simulink model "Control_model_10DOF_fin"  (R2016b)
settings: Solver=FixedStepAuto  StartTime=0.0  StopTime=10  FixedStep=0.0001  RelTol=1e-3
InitFcn:
  | Initialisation_ctr_10DOF_fin
values from neighbouring files (symbols this model uses):
  COM_Parameters = [-lpelvis/2;r2;0]    [Initialisation_ctr_10DOF_fin.m]
  DH_Parameters = [hfoot 0 ... (first row only)    [Initialisation_ctr_10DOF_fin.m]
  dTrunk = trunklbd(3)    [Initialisation_ctr_10DOF_fin.m]
  dxFootSM = dxFoot    [Initialisation_ctr_10DOF_fin.m]
  dxTrunk = 0.1    [Initialisation_ctr_10DOF_fin.m]
  Foot_Parameters = [0;-(lFoot/2-lHeel);0]    [Initialisation_ctr_10DOF_fin.m]
  HAA2HEE = [0; 0; 0.001]    [Initialisation_ctr_10DOF_fin.m]
  HEE2HFE = 0.5*[0.2; 0; 0]    [Initialisation_ctr_10DOF_fin.m]
  height_vrp = CoM_position(1)    [Initialisation_ctr_10DOF_fin.m]
  hTrunk = trunklbd(1)    [Initialisation_ctr_10DOF_fin.m]
  initial_CoM_position = R*CoM_position    [Initialisation_ctr_10DOF_fin.m]
  initial_CoM_velocity = [0;0;0]    [Initialisation_ctr_10DOF_fin.m]
  initial_left_foot = [0;0;-stance_width/2]    [Initialisation_ctr_10DOF_fin.m]
  initial_right_foot = [0;0;stance_width/2]    [Initialisation_ctr_10DOF_fin.m]
  initial_RorL = 0    [Initialisation_ctr_10DOF_fin.m]
  jointsinitial = [9;-15;6;0;0;6;-15;9]/180*pi    [Initialisation_ctr_10DOF_fin.m]
  K_DCM = 4.3*[1 0 0 ... (first row only)    [Initialisation_ctr_10DOF_fin.m]
  kD_left = mbody*[0.95 0 0 0 ... (first row only)    [Initialisation_ctr_10DOF_fin.m]
  kD_right = mbody*[0.12 0 0 0 ... (first row only)    [Initialisation_ctr_10DOF_fin.m]
  kI_left = mbody*[35 0 0 0 ... (first row only)    [Initialisation_ctr_10DOF_fin.m]
  kI_right = mbody*[38.2 0 0 0 ... (first row only)    [Initialisation_ctr_10DOF_fin.m]
  kP_left = mbody*[75 0 0 0 ... (first row only)    [Initialisation_ctr_10DOF_fin.m]
  kP_right = mbody*[5.6 0 0 0 ... (first row only)    [Initialisation_ctr_10DOF_fin.m]
  Lenght = [lShank;lThigh]    [Initialisation_ctr_10DOF_fin.m]
  lFootSM = lFoot    [Initialisation_ctr_10DOF_fin.m]
  lpelvis = wPelvis    [Initialisation_ctr_10DOF_fin.m]
  mass = mbody    (= 60)    [Initialisation_ctr_10DOF_fin.m]
  Masses = [mThigh; mShank; mTrunk]    [Initialisation_ctr_10DOF_fin.m]
  nb_step = 4    [Initialisation_ctr_10DOF_fin.m]
  nb_step_pattern = 20    [Initialisation_ctr_10DOF_fin.m]
  Pelvis_Parameters = [-lpelvis/2;hTrunk/2;0]    [Initialisation_ctr_10DOF_fin.m]
  stance_width = lpelvis    [Initialisation_ctr_10DOF_fin.m]
  stride_lenght = 0.50    (= 0.5)    [Initialisation_ctr_10DOF_fin.m]
  T_DS = time_DS    (= 0.4)    [Initialisation_ctr_10DOF_fin.m]
  T_IT = time_DS    (= 0.4)    [Initialisation_ctr_10DOF_fin.m]
  T_SS = time_swing    (= 1.6)    [Initialisation_ctr_10DOF_fin.m]
  time_DS = (time_stance-time_swing)/2    (= 0.4)    [Initialisation_ctr_10DOF_fin.m]
  time_stance = 60/100*time_stride    (= 2.4)    [Initialisation_ctr_10DOF_fin.m]
  time_step = time_stride/2    (= 2)    [Initialisation_ctr_10DOF_fin.m]
  time_swing = 40/100*time_stride    (= 1.6)    [Initialisation_ctr_10DOF_fin.m]
  validity_angle = [-20*pi/180 20*pi/180 ... (first row only)    [Initialisation_ctr_10DOF_fin.m]
  wTrunk = trunklbd(2)    [Initialisation_ctr_10DOF_fin.m]
  x4CoM = CoM_position(1)-XR4(1)    [Initialisation_ctr_10DOF_fin.m]
undefined symbols (not defined in the file or in its folder): dsegment, hFoot, l, lFoot, omega0_x, omega0_z, rho, wPelvis, X, Xp_x, Xp_z, Y, Z
undefined symbols (not defined in the file): k_grf, lShankSM, lThighSM, mShank, mThigh
libraries: nesl_utility x247, sm_lib x215, dspindex x12, FootPlacementLibrary x8, dspsigops x4, dspswit3 x1
(part 6 of 18)

== system Control_model_10DOF_fin/10DoF Walker SimMechanics Model/Graphic/extrapolated CoM1 ==
  Foot_adjust : Inport
  Cartesian Joint : sm_lib/Joints/Cartesian Joint  SenseConstraintForce=off  SenseConstraintForceX=off  SenseConstraintForceY=off  SenseConstraintForceZ=off  SenseConstraintTorque=off  SenseConstraintTorqueX=off  SenseConstraintTorqueY=off  SenseConstraintTorqueZ=off  SenseTotalForce=off  SenseTotalForceX=off  SenseTotalForceY=off  SenseTotalForceZ=off  SenseTotalTorque=off  SenseTotalTorqueX=off  SenseTotalTorqueY=off  SenseTotalTorqueZ=off  CompositeWrenchDir=FollowerOnBase  CompositeWrenchFrame=BaseFrame  PxEquilibriumPosition=0  PxEquilibriumPositionUnits=m  PxSpringStiffness=0  PxSpringStiffnessUnits=N/m  PxDampingCoefficient=0  PxDampingCoefficientUnits=N/(m/s)  PxTorqueActuationMode=ComputedTorque  PxMotionActuationMode=InputMotion  PxSensePosition=off  PxSenseVelocity=off  PxSenseAcceleration=off  PxSenseTorqueForce=off  PxPositionTargetSpecify=on  PxPositionTargetPriority=Low  PxPositionTargetValue=0  PxPositionTargetValueUnits=m  PxVelocityTargetSpecify=off  PxVelocityTargetPriority=High  PxVelocityTargetValue=0  PxVelocityTargetValueUnits=m/s  PyEquilibriumPosition=0  PyEquilibriumPositionUnits=m  PySpringStiffness=0  PySpringStiffnessUnits=N/m  PyDampingCoefficient=0  PyDampingCoefficientUnits=N/(m/s)  PyTorqueActuationMode=ComputedTorque  PyMotionActuationMode=InputMotion  PySensePosition=off  PySenseVelocity=off  PySenseAcceleration=off  PySenseTorqueForce=off  PyPositionTargetSpecify=on  PyPositionTargetPriority=Low  PyPositionTargetValue=0  PyPositionTargetValueUnits=m  PyVelocityTargetSpecify=off  PyVelocityTargetPriority=High  PyVelocityTargetValue=0  PyVelocityTargetValueUnits=m/s  PzEquilibriumPosition=0  PzEquilibriumPositionUnits=m  PzSpringStiffness=0  PzSpringStiffnessUnits=N/m  PzDampingCoefficient=0  PzDampingCoefficientUnits=N/(m/s)  PzTorqueActuationMode=ComputedTorque  PzMotionActuationMode=InputMotion  PzSensePosition=off  PzSenseVelocity=off  PzSenseAcceleration=off  PzSenseTorqueForce=off  PzPositionTargetSpecify=on  PzPositionTargetPriority=Low  PzPositionTargetValue=0  PzPositionTargetValueUnits=m  PzVelocityTargetSpecify=off  PzVelocityTargetPriority=High  PzVelocityTargetValue=0  PzVelocityTargetValueUnits=m/s
  Demux : Demux  Outputs=3
  Graphic : sm_lib/Body Elements/Graphic  GraphicType=Marker  MarkerShape=Sphere  MarkerSize=10  GraphicVisPropType=SimpleVisualProperties  GraphicDiffuseColor=[0.0 0.2 0.4]  GraphicSpecularColor=[0.5 0.5 0.5 1.0]  GraphicAmbientColor=[0.15 0.15 0.15 1.0]  GraphicEmissiveColor=[0.0 0.0 0.0 1.0]  GraphicShininess=75  GraphicOpacity=1.0
  Memory2 : Memory  X0=[0;0;0]
  Rigid Transform1 : sm_lib/Frames and Transforms/Rigid Transform  TranslationMethod=None  TranslationStandardOffset=0  TranslationLengthUnit=m  TranslationStandardAxis=+Z  TranslationCartesianOffset=[0 0 0]  TranslationROffset=0  TranslationROffsetUnits=m  TranslationZOffset=0  TranslationZOffsetUnits=m  TranslationThetaOffset=0  TranslationThetaOffsetUnits=deg  RotationMethod=None  RotationAngleUnits=deg  RotationStandardAxis=+Z  RotationAngle=0.0  RotationArbitraryAxis=[0 0 1]  FollAlignAxisA=+X  BaseAlignAxisA=+Y  FollAlignAxisB=+Y  BaseAlignAxisB=+Z  RotationSequenceAxes=FollowerAxes  RotationSequence=XYX  RotationSequenceAngles=[0 0 0]  RotationSequenceAnglesUnits=deg  RotationMatrix=[1 0 0; 0 1 0; 0 0 1]
  Simulink-PS Converter1 : nesl_utility/Simulink-PS Converter  PhysicalDomain=network_engine_domain  SubClassName=ps_input  LeftPortType=input  RightPortType=output  PseudoPeriodic=off  Frequencies=[]  NoiseDistribution=none  NoiseParameters=[]  Unit=m  AffineConversion=on  InputFiltering=off  SimscapeFilterOrder=1  InputFilterTimeConstant=0.001  UdotUserProvided=1
  Simulink-PS Converter2 : nesl_utility/Simulink-PS Converter  PhysicalDomain=network_engine_domain  SubClassName=ps_input  LeftPortType=input  RightPortType=output  PseudoPeriodic=off  Frequencies=[]  NoiseDistribution=none  NoiseParameters=[]  Unit=m  AffineConversion=on  InputFiltering=off  SimscapeFilterOrder=1  InputFilterTimeConstant=0.001  UdotUserProvided=1
  Simulink-PS Converter7 : nesl_utility/Simulink-PS Converter  PhysicalDomain=network_engine_domain  SubClassName=ps_input  LeftPortType=input  RightPortType=output  PseudoPeriodic=off  Frequencies=[]  NoiseDistribution=none  NoiseParameters=[]  Unit=m  AffineConversion=on  InputFiltering=off  SimscapeFilterOrder=1  InputFilterTimeConstant=0.001  UdotUserProvided=1
  Base : PMIOPort  Port=1  Side=Left
  wires:
  Demux/1 -> Simulink-PS Converter7/1
  Demux/2 -> Simulink-PS Converter1/1
  Demux/3 -> Simulink-PS Converter2/1
  Memory2/1 -> Demux/1
  Foot_adjust/1 -> Memory2/1
  connections:
  Rigid Transform1/LConn1 -- Cartesian Joint/RConn1
  Simulink-PS Converter7/RConn1 -- Cartesian Joint/LConn2
  Rigid Transform1/RConn1 -- Graphic/RConn1
  Simulink-PS Converter1/RConn1 -- Cartesian Joint/LConn3
  Simulink-PS Converter2/RConn1 -- Cartesian Joint/LConn4
  Base/RConn1 -- Cartesian Joint/LConn1

== system Control_model_10DOF_fin/10DoF Walker SimMechanics Model/trunk/Forward Initial Velocity ==
  PelvisForceVector : Inport
  Perturbation : Inport  Port=2
  6-DOF Joint : sm_lib/Joints/6-DOF Joint  SenseConstraintForce=off  SenseConstraintForceX=off  SenseConstraintForceY=off  SenseConstraintForceZ=off  SenseConstraintTorque=off  SenseConstraintTorqueX=off  SenseConstraintTorqueY=off  SenseConstraintTorqueZ=off  SenseTotalForce=off  SenseTotalForceX=off  SenseTotalForceY=off  SenseTotalForceZ=off  SenseTotalTorque=off  SenseTotalTorqueX=off  SenseTotalTorqueY=off  SenseTotalTorqueZ=off  CompositeWrenchDir=FollowerOnBase  CompositeWrenchFrame=BaseFrame  PxEquilibriumPosition=0  PxEquilibriumPositionUnits=m  PxSpringStiffness=0  PxSpringStiffnessUnits=N/m  PxDampingCoefficient=0  PxDampingCoefficientUnits=N/(m/s)  PxTorqueActuationMode=NoTorque  PxMotionActuationMode=ComputedMotion  PxSensePosition=off  PxSenseVelocity=off  PxSenseAcceleration=off  PxSenseTorqueForce=off  PxPositionTargetSpecify=off  PxPositionTargetPriority=High  PxPositionTargetValue=0  PxPositionTargetValueUnits=m  PxVelocityTargetSpecify=off  PxVelocityTargetPriority=Low  PxVelocityTargetValue=initial_CoM_velocity(1)  PxVelocityTargetValueUnits=m/s  PyEquilibriumPosition=0  PyEquilibriumPositionUnits=m  PySpringStiffness=0  PySpringStiffnessUnits=N/m  PyDampingCoefficient=0  PyDampingCoefficientUnits=N/(m/s)  PyTorqueActuationMode=NoTorque  PyMotionActuationMode=ComputedMotion  PySensePosition=off  PySenseVelocity=off  PySenseAcceleration=off  PySenseTorqueForce=off  PyPositionTargetSpecify=off  PyPositionTargetPriority=High  PyPositionTargetValue=0  PyPositionTargetValueUnits=m  PyVelocityTargetSpecify=off  PyVelocityTargetPriority=Low  PyVelocityTargetValue=initial_CoM_velocity(2)  PyVelocityTargetValueUnits=m/s  PzEquilibriumPosition=0  PzEquilibriumPositionUnits=m  PzSpringStiffness=0  PzSpringStiffnessUnits=N/m  PzDampingCoefficient=0  PzDampingCoefficientUnits=N/(m/s)  PzTorqueActuationMode=NoTorque  PzMotionActuationMode=ComputedMotion  PzSensePosition=off  PzSenseVelocity=off  PzSenseAcceleration=off  PzSenseTorqueForce=off  PzPositionTargetSpecify=off  PzPositionTargetPriority=High  PzPositionTargetValue=0  PzPositionTargetValueUnits=m  PzVelocityTargetSpecify=off  PzVelocityTargetPriority=Low  PzVelocityTargetValue=initial_CoM_velocity(3)  PzVelocityTargetValueUnits=m/s  SphDefPosRotationMethod=None  SphDefPosRotationAngleUnits=deg  SphDefPosRotationStandardAxis=+Z  SphDefPosRotationAngle=0  SphDefPosRotationArbitraryAxis=[0 0 1]  SphDefPosFollAlignAxisA=+X  SphDefPosBaseAlignAxisA=+Y  SphDefPosFollAlignAxisB=+Y  SphDefPosBaseAlignAxisB=+Z  SphDefPosRotationSequenceAxes=FollowerAxes  SphDefPosRotationSequence=XYX  SphDefPosRotationSequenceAngles=[0 0 0]  SphDefPosRotationSequenceAnglesUnits=deg  SphDefPosRotationMatrix=[1 0 0; 0 1 0; 0 0 1]  SphEqPosRotationMethod=StandardAxis  SphEqPosRotationAngleUnits=deg  SphEqPosRotationStandardAxis=+Y  SphEqPosRotationAngle=0  SphEqPosRotationArbitraryAxis=[0 0 1]  SphEqPosFollAlignAxisA=+X  SphEqPosBaseAlignAxisA=+Y  SphEqPosFollAlignAxisB=+Y  SphEqPosBaseAlignAxisB=+Z  SphEqPosRotationSequenceAxes=FollowerAxes  SphEqPosRotationSequence=XYX  SphEqPosRotationSequenceAngles=[0 0 0]  SphEqPosRotationSequenceAnglesUnits=deg  SphEqPosRotationMatrix=[1 0 0; 0 1 0; 0 0 1]  SphSpringStiffness=100  SphSpringStiffnessUnits=N*m/rad  SphDampingCoefficient=10  SphDampingCoefficientUnits=N*m/(rad/s)  SphActuateTorqueX=off  SphActuateTorqueY=off  SphActuateTorqueZ=off  SphActuateTorque=off  SphTorqueActuationMode=NoTorque  SphMotionActuationMode=ComputedMotion  SphActuationFrame=BaseFrame  SphSensePosition=off  SphSenseVelocityX=off  SphSenseVelocityY=off  SphSenseVelocityZ=off  SphSenseVelocity=off  SphSenseAccelerationX=off  SphSenseAccelerationY=off  SphSenseAccelerationZ=off  SphSenseAcceleration=off  SphSenseTorqueX=off  SphSenseTorqueY=off  SphSenseTorqueZ=off  SphSenseTorqueForce=off  SphSensingFrame=BaseFrame  SphPositionTargetRotationMethod=StandardAxis  SphPositionTargetRotationAngleUnits=deg  SphPositionTargetRotationStandardAxis=+X  SphPositionTargetRotationAngle=0  SphPositionTargetRotationArbitraryAxis=[0 0 1]  SphPositionTargetFollAlignAxisA=+X  SphPositionTargetBaseAlignAxisA=+Y  SphPositionTargetFollAlignAxisB=+Y  SphPositionTargetBaseAlignAxisB=+Z  SphPositionTargetRotationSequenceAxes=FollowerAxes  SphPositionTargetRotationSequence=XYX  SphPositionTargetRotationSequenceAngles=[0 0 0]  SphPositionTargetRotationSequenceAnglesUnits=deg  SphPositionTargetRotationMatrix=[1 0 0; 0 1 0; 0 0 1]  SphPositionTargetSpecify=off  SphPositionTargetPriority=Low  SphVelocityTargetValue=[0 0 0]  SphVelocityTargetValueUnits=deg/s  SphVelocityTargetSpecify=off  SphVelocityTargetPriority=High  SphVelocityTargetInFollowerFrame=on
  Demux : Demux  Outputs=3
  External Force  and Torque : sm_lib/Forces and Torques/External Force and Torque  ForceResolutionFrame=World  EnableForceX=off  EnableForceY=off  EnableForceZ=on  EnableForce=off  TorqueResolutionFrame=AttachedFrame  EnableTorqueX=off  EnableTorqueY=off  EnableTorqueZ=off  EnableTorque=off
  External Force  and Torque2 : sm_lib/Forces and Torques/External Force and Torque  ForceResolutionFrame=World  EnableForceX=on  EnableForceY=off  EnableForceZ=on  EnableForce=off  TorqueResolutionFrame=AttachedFrame  EnableTorqueX=off  EnableTorqueY=off  EnableTorqueZ=off  EnableTorque=off
  Mux : Mux  Inputs=3
  Mux1 : Mux  Inputs=3
  PS-Simulink Converter{1..7} (7 alike) : nesl_utility/PS-Simulink Converter  PhysicalDomain=network_engine_domain  SubClassName=ps_output  LeftPortType=input  RightPortType=output  PseudoPeriodic=off  Frequencies=[]  Unit=1  AffineConversion=off
  Simulink-PS Converter1 : nesl_utility/Simulink-PS Converter  PhysicalDomain=network_engine_domain  SubClassName=ps_input  LeftPortType=input  RightPortType=output  PseudoPeriodic=off  Frequencies=[]  NoiseDistribution=none  NoiseParameters=[]  Unit=N  AffineConversion=off  InputFiltering=off  SimscapeFilterOrder=1  InputFilterTimeConstant=0.001  UdotUserProvided=1
  Simulink-PS Converter3 : nesl_utility/Simulink-PS Converter  PhysicalDomain=network_engine_domain  SubClassName=ps_input  LeftPortType=input  RightPortType=output  PseudoPeriodic=off  Frequencies=[]  NoiseDistribution=none  NoiseParameters=[]  Unit=N  AffineConversion=off  InputFiltering=off  SimscapeFilterOrder=1  InputFilterTimeConstant=0.001  UdotUserProvided=1
  Terminator : Terminator
  Terminator1 : Terminator
  Transform  Sensor : sm_lib/Frames and Transforms/Transform Sensor  MeasurementFrame=Base  SenseAngle=off  SenseAxis=off  SenseAngle1=off  SenseAngle2=off  SenseAngle3=off  SenseQ=off  SenseR=off  SenseOmegaX=off  SenseOmegaY=off  SenseOmegaZ=off  SenseOmega1=off  SenseOmega2=off  SenseOmega3=off  SenseQDot=off  SenseRDot=off  SenseAlphaX=off  SenseAlphaY=off  SenseAlphaZ=off  SenseAlpha1=off  SenseAlpha2=off  SenseAlpha3=off  SenseQDDot=off  SenseRDDot=off  SenseX=off  SenseY=off  SenseZ=off  SenseRad=off  SenseAzim=off  SenseDist=off  SenseInc=off  SenseXDot=off  SenseYDot=off  SenseZDot=off  SenseRadDot=off  SenseAzimDot=off  SenseDistDot=off  SenseIncDot=off  SenseXDDot=on  SenseYDDot=on  SenseZDDot=on  SenseRadDDot=off  SenseAzimDDot=off  SenseDistDDot=off  SenseIncDDot=off
  Transform  Sensor1 : sm_lib/Frames and Transforms/Transform Sensor  MeasurementFrame=Base  SenseAngle=off  SenseAxis=off  SenseAngle1=off  SenseAngle2=off  SenseAngle3=off  SenseQ=off  SenseR=off  SenseOmegaX=off  SenseOmegaY=off  SenseOmegaZ=off  SenseOmega1=off  SenseOmega2=off  SenseOmega3=off  SenseQDot=off  SenseRDot=off  SenseAlphaX=off  SenseAlphaY=off  SenseAlphaZ=off  SenseAlpha1=off  SenseAlpha2=off  SenseAlpha3=off  SenseQDDot=off  SenseRDDot=off  SenseX=off  SenseY=off  SenseZ=off  SenseRad=off  SenseAzim=off  SenseDist=off  SenseInc=off  SenseXDot=on  SenseYDot=on  SenseZDot=on  SenseRadDot=off  SenseAzimDot=off  SenseDistDot=off  SenseIncDot=off  SenseXDDot=off  SenseYDDot=off  SenseZDDot=off  SenseRadDDot=off  SenseAzimDDot=off  SenseDistDDot=off  SenseIncDDot=off
  Transform  Sensor2 : sm_lib/Frames and Transforms/Transform Sensor  MeasurementFrame=World  SenseAngle=off  SenseAxis=off  SenseAngle1=off  SenseAngle2=off  SenseAngle3=off  SenseQ=off  SenseR=on  SenseOmegaX=off  SenseOmegaY=off  SenseOmegaZ=off  SenseOmega1=off  SenseOmega2=off  SenseOmega3=off  SenseQDot=off  SenseRDot=off  SenseAlphaX=off  SenseAlphaY=off  SenseAlphaZ=off  SenseAlpha1=off  SenseAlpha2=off  SenseAlpha3=off  SenseQDDot=off  SenseRDDot=off  SenseX=off  SenseY=off  SenseZ=off  SenseRad=off  SenseAzim=off  SenseDist=off  SenseInc=off  SenseXDot=off  SenseYDot=off  SenseZDot=off  SenseRadDot=off  SenseAzimDot=off  SenseDistDot=off  SenseIncDot=off  SenseXDDot=off  SenseYDDot=off  SenseZDDot=off  SenseRadDDot=off  SenseAzimDDot=off  SenseDistDDot=off  SenseIncDDot=off
  World : PMIOPort  Port=1  Side=Right
  PelvisCentre : PMIOPort  Port=2  Side=Right
  A_CoM : Outport
  V_CoM : Outport  Port=2
  Rtrunk : Outport  Port=3
  wires:
  PelvisForceVector/1 -> Demux/1
  PS-Simulink Converter3/1 -> Mux/1
  Mux/1 -> A_CoM/1
  PS-Simulink Converter1/1 -> Mux/2
  PS-Simulink Converter2/1 -> Mux/3
  PS-Simulink Converter4/1 -> Mux1/1
  Mux1/1 -> V_CoM/1
  PS-Simulink Converter5/1 -> Mux1/2
  PS-Simulink Converter6/1 -> Mux1/3
  PS-Simulink Converter7/1 -> Rtrunk/1
  Demux/3 -> Simulink-PS Converter1/1
  Perturbation/1 -> Simulink-PS Converter3/1
  Demux/1 -> Terminator/1
  Demux/2 -> Terminator1/1
  connections:
  6-DOF Joint/LConn1 -- Transform  Sensor1/LConn1 -- Transform  Sensor/LConn1 -- Transform  Sensor2/LConn1 -- World/RConn1
  6-DOF Joint/RConn1 -- Transform  Sensor2/RConn1 -- External Force  and Torque2/RConn1 -- External Force  and Torque/RConn1 -- Transform  Sensor1/RConn1 -- Transform  Sensor/RConn1 -- PelvisCentre/RConn1
  PS-Simulink Converter3/LConn1 -- Transform  Sensor/RConn2
  Simulink-PS Converter1/RConn1 -- External Force  and Torque/LConn1
  Transform  Sensor/RConn3 -- PS-Simulink Converter1/LConn1
  PS-Simulink Converter2/LConn1 -- Transform  Sensor/RConn4
  PS-Simulink Converter4/LConn1 -- Transform  Sensor1/RConn2
  PS-Simulink Converter5/LConn1 -- Transform  Sensor1/RConn3
  PS-Simulink Converter6/LConn1 -- Transform  Sensor1/RConn4
  PS-Simulink Converter7/LConn1 -- Transform  Sensor2/RConn2
  Simulink-PS Converter3/RConn1 -- External Force  and Torque2/LConn1

== system Control_model_10DOF_fin/10DoF Walker SimMechanics Model/trunk/Scope x3 ==
  Input : Inport
  Demux : Demux  Outputs=3
  Scope1 : Scope
  Scope2 : Scope
  Scope3 : Scope
  wires:
  Input/1 -> Demux/1
  Demux/2 -> Scope1/1
  Demux/3 -> Scope2/1
  Demux/1 -> Scope3/1

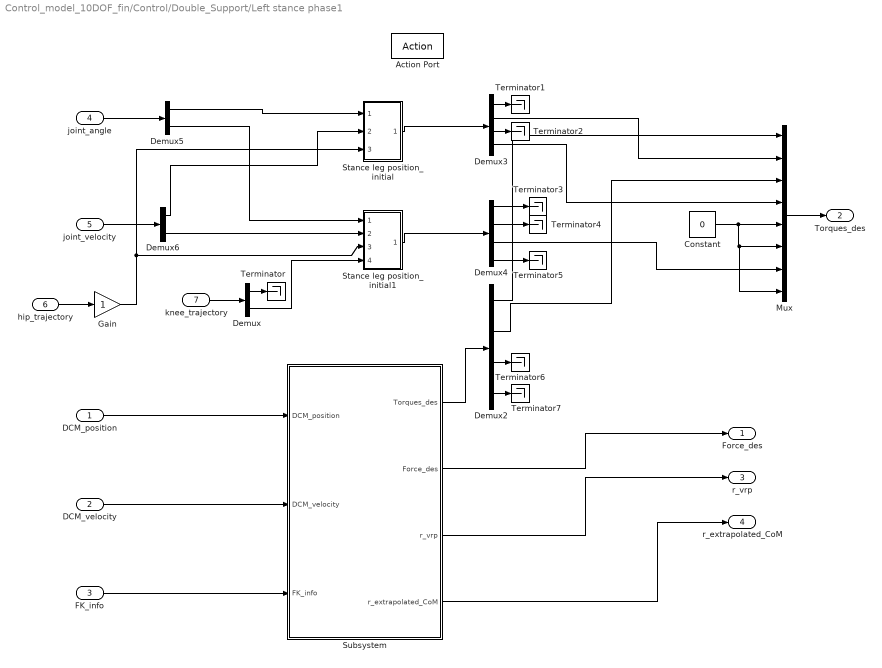
== system Control_model_10DOF_fin/Control/Double_Support/Left stance phase1 ==
  DCM_position : Inport
  DCM_velocity : Inport  Port=2
  FK_info : Inport  Port=3
  joint_angle : Inport  Port=4
  joint_velocity : Inport  Port=5
  hip_trajectory : Inport  Port=6
  knee_trajectory : Inport  Port=7
  Action Port : ActionPort  ActionType=else
  Constant : Constant  Value=0
  Demux : Demux  Outputs=2
  Demux2 : Demux
  Demux3 : Demux
  Demux4 : Demux
  Demux5 : Demux  Outputs=2
  Demux6 : Demux  Outputs=2
  Gain : Gain
  Mux : Mux  Inputs=8
  Stance leg position_initial : Subsystem
  Stance leg position_initial1 : Subsystem
  Subsystem : Subsystem
  Terminator{,1..7} (8 alike) : Terminator
  Force_des : Outport
  Torques_des : Outport  Port=2  OutDataTypeStr=double  Unit=N*m
  r_vrp : Outport  Port=3
  r_extrapolated_CoM : Outport  Port=4
  wires:
  joint_angle/1 -> Demux5/1
  joint_velocity/1 -> Demux6/1
  Subsystem/1(Torques_des) -> Demux2/1
  Mux/1 -> Torques_des/1
  Stance leg position_initial/1(torques) -> Demux3/1
  Stance leg position_initial1/1(torques) -> Demux4/1
  Demux5/1 -> Stance leg position_initial/1(position)
  Demux5/2 -> Stance leg position_initial1/1(position)
  Demux6/2 -> Stance leg position_initial1/2(velocity)
  Demux6/1 -> Stance leg position_initial/2(velocity)
  Subsystem/2(Force_des) -> Force_des/1
  Subsystem/3(r_vrp) -> r_vrp/1
  Subsystem/4(r_extrapolated_CoM) -> r_extrapolated_CoM/1
  Demux3/2 -> Mux/2
  Demux3/4 -> Mux/4
  DCM_position/1 -> Subsystem/1(DCM_position)
  FK_info/1 -> Subsystem/3(FK_info)
  DCM_velocity/1 -> Subsystem/2(DCM_velocity)
  hip_trajectory/1 -> Gain/1
  Gain/1 -> Stance leg position_initial/3(theta4), Stance leg position_initial1/3(theta5)
  Demux2/2 -> Mux/3
  Demux2/1 -> Mux/1
  Demux4/3 -> Mux/7
  knee_trajectory/1 -> Demux/1
  Demux/2 -> Stance leg position_initial1/4(knee_trajectory)
  Demux/1 -> Terminator/1
  Demux3/1 -> Terminator1/1
  Demux3/3 -> Terminator2/1
  Demux4/1 -> Terminator3/1
  Demux4/2 -> Terminator4/1
  Demux4/4 -> Terminator5/1
  Demux2/3 -> Terminator6/1
  Demux2/4 -> Terminator7/1
  Constant/1 -> Mux/8, Mux/6, Mux/5

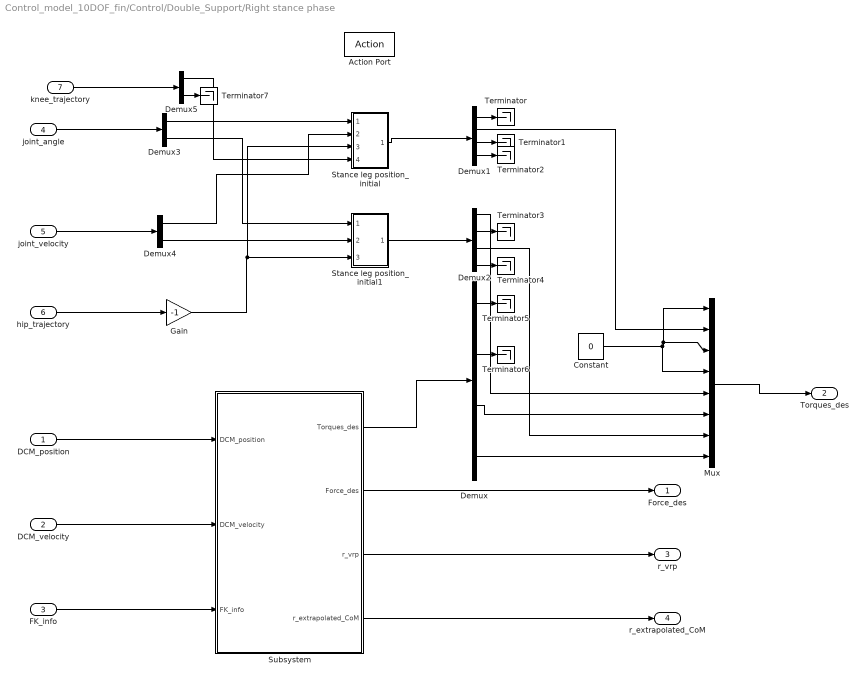
== system Control_model_10DOF_fin/Control/Double_Support/Right stance phase ==
  DCM_position : Inport
  DCM_velocity : Inport  Port=2
  FK_info : Inport  Port=3
  joint_angle : Inport  Port=4
  joint_velocity : Inport  Port=5
  hip_trajectory : Inport  Port=6
  knee_trajectory : Inport  Port=7
  Action Port : ActionPort  ActionType=then
  Constant : Constant  Value=0
  Demux : Demux
  Demux1 : Demux
  Demux2 : Demux
  Demux3 : Demux  Outputs=2
  Demux4 : Demux  Outputs=2
  Demux5 : Demux  Outputs=2
  Gain : Gain  Gain=-1
  Mux : Mux  Inputs=8
  Stance leg position_initial : Subsystem
  Stance leg position_initial1 : Subsystem
  Subsystem : Subsystem
  Terminator{,1..7} (8 alike) : Terminator
  Force_des : Outport
  Torques_des : Outport  Port=2  OutDataTypeStr=double  Unit=N*m
  r_vrp : Outport  Port=3
  r_extrapolated_CoM : Outport  Port=4
  wires:
  DCM_position/1 -> Subsystem/1(DCM_position)
  DCM_velocity/1 -> Subsystem/2(DCM_velocity)
  FK_info/1 -> Subsystem/3(FK_info)
  Subsystem/2(Force_des) -> Force_des/1
  Subsystem/3(r_vrp) -> r_vrp/1
  Subsystem/4(r_extrapolated_CoM) -> r_extrapolated_CoM/1
  Subsystem/1(Torques_des) -> Demux/1
  Stance leg position_initial/1(torques) -> Demux1/1
  Mux/1 -> Torques_des/1
  Stance leg position_initial1/1(torques) -> Demux2/1
  Demux3/1 -> Stance leg position_initial/1(position)
  Demux3/2 -> Stance leg position_initial1/1(position)
  Demux4/2 -> Stance leg position_initial1/2(velocity)
  Demux4/1 -> Stance leg position_initial/2(velocity)
  joint_angle/1 -> Demux3/1
  joint_velocity/1 -> Demux4/1
  Demux2/3 -> Mux/7
  Demux2/1 -> Mux/5
  Demux/3 -> Mux/6
  Demux/4 -> Mux/8
  hip_trajectory/1 -> Gain/1
  Gain/1 -> Stance leg position_initial/3(theta4), Stance leg position_initial1/3(theta5)
  knee_trajectory/1 -> Demux5/1
  Demux5/1 -> Stance leg position_initial/4(knee_trajectory)
  Demux1/2 -> Mux/2
  Demux1/1 -> Terminator/1
  Demux1/3 -> Terminator1/1
  Demux1/4 -> Terminator2/1
  Demux2/2 -> Terminator3/1
  Demux2/4 -> Terminator4/1
  Demux/1 -> Terminator5/1
  Demux/2 -> Terminator6/1
  Constant/1 -> Mux/4, Mux/3, Mux/1
  Demux5/2 -> Terminator7/1

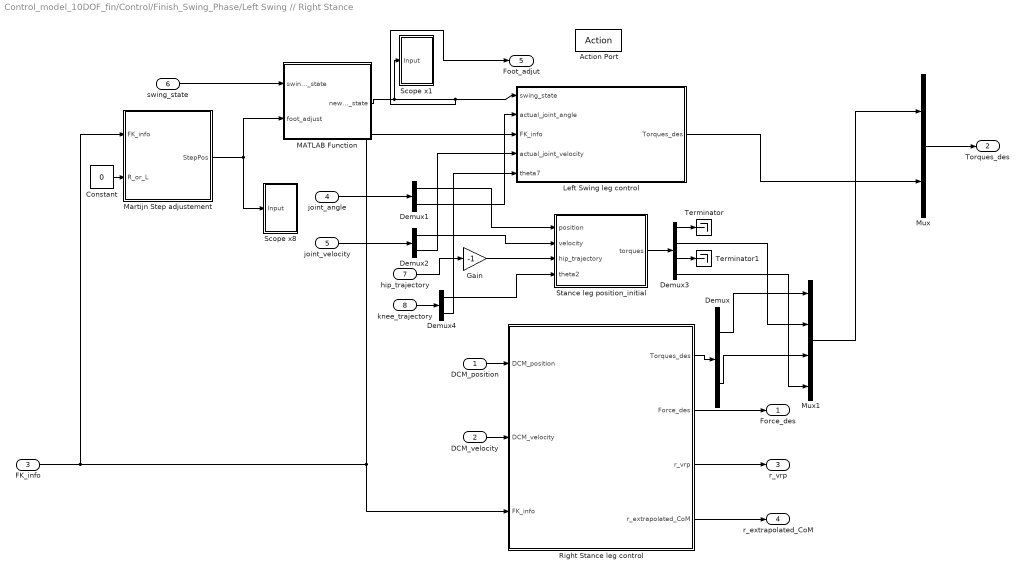
== system Control_model_10DOF_fin/Control/Finish_Swing_Phase/Left Swing // Right Stance ==
  DCM_position : Inport
  DCM_velocity : Inport  Port=2
  FK_info : Inport  Port=3
  joint_angle : Inport  Port=4
  joint_velocity : Inport  Port=5
  swing_state : Inport  Port=6
  hip_trajectory : Inport  Port=7
  knee_trajectory : Inport  Port=8
  Action Port : ActionPort  ActionType=then
  Constant : Constant  Value=0
  Demux{,1..2,4} (4 alike) : Demux  Outputs=2
  Demux3 : Demux
  Gain : Gain  Gain=-1
  Left Swing leg control : Subsystem
  MATLAB Function : MATLAB Function  TreatAsAtomicUnit=on
  Martijn Step adjustement : Subsystem
  Mux : Mux  Inputs=2
  Mux1 : Mux
  Right Stance leg control : Subsystem
  Scope x1 : Subsystem
  Scope x8 : Subsystem
  Stance leg position_initial : Subsystem
  Terminator : Terminator
  Terminator1 : Terminator
  Force_des : Outport
  Torques_des : Outport  Port=2  OutDataTypeStr=double  Unit=N*m
  r_vrp : Outport  Port=3
  r_extrapolated_CoM : Outport  Port=4
  Foot_adjut : Outport  Port=5
  wires:
  Left Swing leg control/1(Torques_des) -> Mux/2
  Right Stance leg control/1(Torques_des) -> Demux/1
  Stance leg position_initial/1(torques) -> Demux3/1
  Demux3/2 -> Mux1/2
  Right Stance leg control/2(Force_des) -> Force_des/1
  Mux/1 -> Torques_des/1
  Right Stance leg control/4(r_extrapolated_CoM) -> r_extrapolated_CoM/1
  Right Stance leg control/3(r_vrp) -> r_vrp/1
  FK_info/1 -> Left Swing leg control/3(FK_info), Right Stance leg control/3(FK_info), Martijn Step adjustement/1(FK_info)
  DCM_velocity/1 -> Right Stance leg control/2(DCM_velocity)
  DCM_position/1 -> Right Stance leg control/1(DCM_position)
  Demux1/1 -> Stance leg position_initial/1(position)
  Demux1/2 -> Left Swing leg control/2(actual_joint_angle)
  joint_angle/1 -> Demux1/1
  joint_velocity/1 -> Demux2/1
  Demux2/1 -> Stance leg position_initial/2(velocity)
  Demux2/2 -> Left Swing leg control/4(actual_joint_velocity)
  Mux1/1 -> Mux/1
  Demux/1 -> Mux1/1
  Demux/2 -> Mux1/3
  Constant/1 -> Martijn Step adjustement/2(R_or_L)
  Martijn Step adjustement/1(StepPos) -> MATLAB Function/2(foot_adjust), Scope x8/1(Input)
  swing_state/1 -> MATLAB Function/1(swing_state)
  MATLAB Function/1(new_swing_state) -> Scope x1/1(Input), Foot_adjut/1, Left Swing leg control/1(swing_state)
  Demux3/4 -> Mux1/4
  hip_trajectory/1 -> Gain/1
  Gain/1 -> Stance leg position_initial/3(hip_trajectory)
  knee_trajectory/1 -> Demux4/1
  Demux4/1 -> Stance leg position_initial/4(theta2)
  Demux4/2 -> Left Swing leg control/5(theta7)
  Demux3/1 -> Terminator/1
  Demux3/3 -> Terminator1/1

== system Control_model_10DOF_fin/Control/Finish_Swing_Phase/Right Swing // Left Stance1 ==
  DCM_position : Inport
  DCM_velocity : Inport  Port=2
  FK_info : Inport  Port=3
  joint_angle : Inport  Port=4
  joint_velocity : Inport  Port=5
  swing_state : Inport  Port=6
  hip_trajectory : Inport  Port=7
  knee_trajectory : Inport  Port=8
  Action Port : ActionPort  ActionType=else
  Constant : Constant
  Demux{,1..2,4} (4 alike) : Demux  Outputs=2
  Demux3 : Demux
  MATLAB Function : MATLAB Function  TreatAsAtomicUnit=on
  Martijn Step adjustement : Subsystem
  Mux : Mux  Inputs=2
  Mux1 : Mux
  Right Swing leg control : Subsystem
  Stance leg control : Subsystem
  Stance leg position_initial1 : Subsystem
  Terminator : Terminator
  Terminator1 : Terminator
  Force_des : Outport
  Torques_des : Outport  Port=2  OutDataTypeStr=double  Unit=N*m
  r_vrp : Outport  Port=3
  r_extrapolated_CoM : Outport  Port=4
  Foot_adjust : Outport  Port=5
  wires:
  Stance leg control/2(Force_des) -> Force_des/1
  Stance leg control/4(r_extrapolated_CoM) -> r_extrapolated_CoM/1
  Stance leg control/3(r_vrp) -> r_vrp/1
  Stance leg control/1(Torques_des) -> Demux/1
  Mux1/1 -> Mux/2
  Mux/1 -> Torques_des/1
  Right Swing leg control/1(Torques_des) -> Mux/1
  DCM_position/1 -> Stance leg control/1(DCM_position)
  DCM_velocity/1 -> Stance leg control/2(DCM_velocity)
  joint_angle/1 -> Demux1/1
  joint_velocity/1 -> Demux2/1
  Demux1/1 -> Right Swing leg control/2(actual_joint_angle)
  Demux1/2 -> Stance leg position_initial1/1(position)
  Demux2/1 -> Right Swing leg control/4(actual_joint_velocity)
  FK_info/1 -> Martijn Step adjustement/1(FK_info), Right Swing leg control/3(FK_info), Stance leg control/3(FK_info)
  Demux2/2 -> Stance leg position_initial1/2(velocity)
  Stance leg position_initial1/1(torques) -> Demux3/1
  Demux3/3 -> Mux1/3
  Demux/2 -> Mux1/4
  Demux/1 -> Mux1/2
  Demux3/1 -> Mux1/1
  hip_trajectory/1 -> Stance leg position_initial1/3(hip_trajectory)
  Constant/1 -> Martijn Step adjustement/2(R_or_L)
  swing_state/1 -> MATLAB Function/1(swing_state)
  Martijn Step adjustement/1(StepPos) -> MATLAB Function/2(foot_adjust)
  MATLAB Function/1(new_swing_state) -> Foot_adjust/1, Right Swing leg control/1(swing_state)
  knee_trajectory/1 -> Demux4/1
  Demux4/1 -> Right Swing leg control/5(theta2)
  Demux4/2 -> Stance leg position_initial1/4(theta7)
  Demux3/2 -> Terminator/1
  Demux3/4 -> Terminator1/1

== system Control_model_10DOF_fin/Control/Inititial_Transfert/Left stance phase1 ==
  DCM_position : Inport
  DCM_velocity : Inport  Port=2
  FK_info : Inport  Port=3
  joint_angle : Inport  Port=4
  joint_velocity : Inport  Port=5
  hip_trajectory : Inport  Port=6
  Action Port : ActionPort  ActionType=else
  Demux2 : Demux
  Demux3 : Demux
  Demux4 : Demux
  Demux5 : Demux  Outputs=2
  Demux6 : Demux  Outputs=2
  Mux : Mux  Inputs=8
  Stance leg position_initial : Subsystem
  Stance leg position_initial1 : Subsystem
  Subsystem : Subsystem
  Terminator{,1..3} (4 alike) : Terminator
  Force_des : Outport
  Torques_des : Outport  Port=2  OutDataTypeStr=double  Unit=N*m
  r_vrp : Outport  Port=3
  r_extrapolated_CoM : Outport  Port=4
  wires:
  joint_angle/1 -> Demux5/1
  joint_velocity/1 -> Demux6/1
  Subsystem/1(Torques_des) -> Demux2/1
  Mux/1 -> Torques_des/1
  Stance leg position_initial/1(torques) -> Demux3/1
  Stance leg position_initial1/1(torques) -> Demux4/1
  Demux5/1 -> Stance leg position_initial/1(position)
  Demux5/2 -> Stance leg position_initial1/1(position)
  Demux6/2 -> Stance leg position_initial1/2(velocity)
  Demux6/1 -> Stance leg position_initial/2(velocity)
  Subsystem/2(Force_des) -> Force_des/1
  Subsystem/3(r_vrp) -> r_vrp/1
  Subsystem/4(r_extrapolated_CoM) -> r_extrapolated_CoM/1
  Demux3/2 -> Mux/2
  Demux3/4 -> Mux/4
  Demux4/1 -> Mux/5
  Demux4/3 -> Mux/7
  Demux2/1 -> Mux/1
  Demux2/2 -> Mux/3
  Demux2/3 -> Mux/6
  Demux2/4 -> Mux/8
  DCM_position/1 -> Subsystem/1(DCM_position)
  FK_info/1 -> Subsystem/3(FK_info)
  DCM_velocity/1 -> Subsystem/2(DCM_velocity)
  hip_trajectory/1 -> Stance leg position_initial/3(theta4), Stance leg position_initial1/3(theta5)
  Demux3/1 -> Terminator/1
  Demux3/3 -> Terminator1/1
  Demux4/2 -> Terminator2/1
  Demux4/4 -> Terminator3/1

== system Control_model_10DOF_fin/Control/Inititial_Transfert/Right stance phase ==
  DCM_position : Inport
  DCM_velocity : Inport  Port=2
  FK_info : Inport  Port=3
  joint_angle : Inport  Port=4
  joint_velocity : Inport  Port=5
  hip_trajectory : Inport  Port=6
  Action Port : ActionPort  ActionType=then
  Demux : Demux
  Demux1 : Demux
  Demux2 : Demux
  Demux3 : Demux  Outputs=2
  Demux4 : Demux  Outputs=2
  Gain : Gain  Gain=-1
  Mux : Mux  Inputs=8
  Stance leg position_initial : Subsystem
  Stance leg position_initial1 : Subsystem
  Subsystem : Subsystem
  Terminator{,1..3} (4 alike) : Terminator
  Force_des : Outport
  Torques_des : Outport  Port=2  OutDataTypeStr=double  Unit=N*m
  r_vrp : Outport  Port=3
  r_extrapolated_CoM : Outport  Port=4
  wires:
  DCM_position/1 -> Subsystem/1(DCM_position)
  DCM_velocity/1 -> Subsystem/2(DCM_velocity)
  FK_info/1 -> Subsystem/3(FK_info)
  Subsystem/2(Force_des) -> Force_des/1
  Subsystem/3(r_vrp) -> r_vrp/1
  Subsystem/4(r_extrapolated_CoM) -> r_extrapolated_CoM/1
  Subsystem/1(Torques_des) -> Demux/1
  Stance leg position_initial/1(torques) -> Demux1/1
  Mux/1 -> Torques_des/1
  Stance leg position_initial1/1(torques) -> Demux2/1
  Demux3/1 -> Stance leg position_initial/1(position)
  Demux3/2 -> Stance leg position_initial1/1(position)
  Demux4/2 -> Stance leg position_initial1/2(velocity)
  Demux4/1 -> Stance leg position_initial/2(velocity)
  joint_angle/1 -> Demux3/1
  joint_velocity/1 -> Demux4/1
  Demux1/2 -> Mux/2
  Demux2/3 -> Mux/7
  Demux1/4 -> Mux/4
  Demux2/1 -> Mux/5
  Demux/1 -> Mux/1
  Demux/2 -> Mux/3
  Demux/3 -> Mux/6
  Demux/4 -> Mux/8
  hip_trajectory/1 -> Gain/1
  Gain/1 -> Stance leg position_initial/3(theta4), Stance leg position_initial1/3(theta5)
  Demux1/1 -> Terminator/1
  Demux1/3 -> Terminator1/1
  Demux2/2 -> Terminator2/1
  Demux2/4 -> Terminator3/1

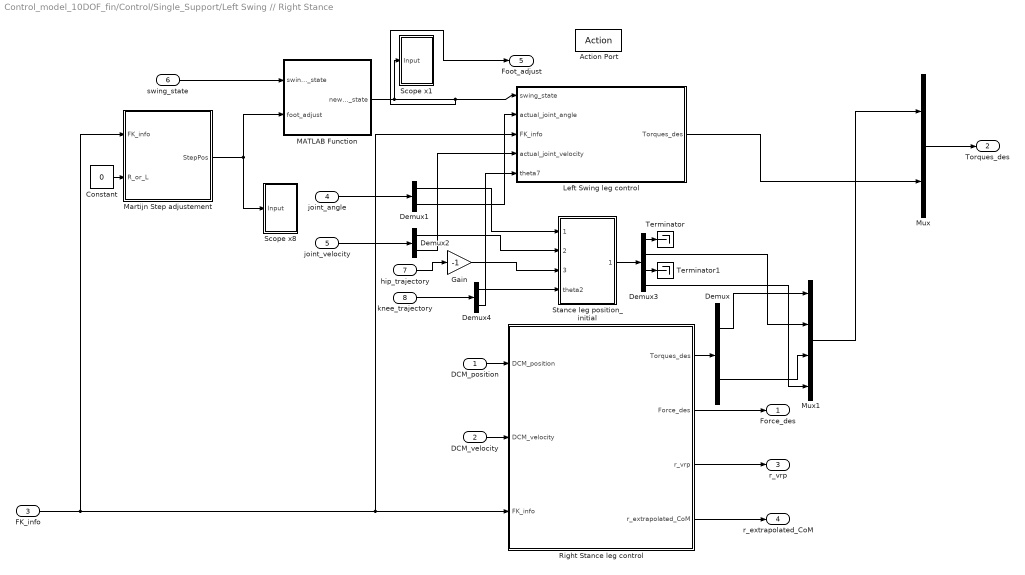
== system Control_model_10DOF_fin/Control/Single_Support/Left Swing // Right Stance ==
  DCM_position : Inport
  DCM_velocity : Inport  Port=2
  FK_info : Inport  Port=3
  joint_angle : Inport  Port=4
  joint_velocity : Inport  Port=5
  swing_state : Inport  Port=6
  hip_trajectory : Inport  Port=7
  knee_trajectory : Inport  Port=8
  Action Port : ActionPort  ActionType=then
  Constant : Constant  Value=0
  Demux{,1..2,4} (4 alike) : Demux  Outputs=2
  Demux3 : Demux
  Gain : Gain  Gain=-1
  Left Swing leg control : Subsystem
  MATLAB Function : MATLAB Function  TreatAsAtomicUnit=on
  Martijn Step adjustement : Subsystem
  Mux : Mux  Inputs=2
  Mux1 : Mux
  Right Stance leg control : Subsystem
  Scope x1 : Subsystem
  Scope x8 : Subsystem
  Stance leg position_initial : Subsystem
  Terminator : Terminator
  Terminator1 : Terminator
  Force_des : Outport
  Torques_des : Outport  Port=2  OutDataTypeStr=double  Unit=N*m
  r_vrp : Outport  Port=3
  r_extrapolated_CoM : Outport  Port=4
  Foot_adjust : Outport  Port=5
  wires:
  Left Swing leg control/1(Torques_des) -> Mux/2
  Right Stance leg control/1(Torques_des) -> Demux/1
  Stance leg position_initial/1(torques) -> Demux3/1
  Demux3/2 -> Mux1/2
  Right Stance leg control/2(Force_des) -> Force_des/1
  Mux/1 -> Torques_des/1
  Right Stance leg control/4(r_extrapolated_CoM) -> r_extrapolated_CoM/1
  Right Stance leg control/3(r_vrp) -> r_vrp/1
  FK_info/1 -> Martijn Step adjustement/1(FK_info), Left Swing leg control/3(FK_info), Right Stance leg control/3(FK_info)
  DCM_velocity/1 -> Right Stance leg control/2(DCM_velocity)
  DCM_position/1 -> Right Stance leg control/1(DCM_position)
  Demux1/1 -> Stance leg position_initial/1(position)
  Demux1/2 -> Left Swing leg control/2(actual_joint_angle)
  joint_angle/1 -> Demux1/1
  joint_velocity/1 -> Demux2/1
  Demux2/1 -> Stance leg position_initial/2(velocity)
  Demux2/2 -> Left Swing leg control/4(actual_joint_velocity)
  Mux1/1 -> Mux/1
  Demux/1 -> Mux1/1
  Demux/2 -> Mux1/3
  Constant/1 -> Martijn Step adjustement/2(R_or_L)
  Martijn Step adjustement/1(StepPos) -> MATLAB Function/2(foot_adjust), Scope x8/1(Input)
  swing_state/1 -> MATLAB Function/1(swing_state)
  MATLAB Function/1(new_swing_state) -> Scope x1/1(Input), Foot_adjust/1, Left Swing leg control/1(swing_state)
  hip_trajectory/1 -> Gain/1
  Demux3/4 -> Mux1/4
  Gain/1 -> Stance leg position_initial/3(hip_trajectory)
  knee_trajectory/1 -> Demux4/1
  Demux4/1 -> Stance leg position_initial/4(theta2)
  Demux4/2 -> Left Swing leg control/5(theta7)
  Demux3/1 -> Terminator/1
  Demux3/3 -> Terminator1/1

== system Control_model_10DOF_fin/Control/Single_Support/Right Swing // Left Stance ==
  DCM_position : Inport
  DCM_velocity : Inport  Port=2
  FK_info : Inport  Port=3
  joint_angle : Inport  Port=4
  joint_velocity : Inport  Port=5
  swing_state : Inport  Port=6
  hip_trajectory : Inport  Port=7
  knee_trajectory : Inport  Port=8
  Action Port : ActionPort  ActionType=else
  Constant : Constant
  Demux{,1..2,4} (4 alike) : Demux  Outputs=2
  Demux3 : Demux
  MATLAB Function : MATLAB Function  TreatAsAtomicUnit=on
  Martijn Step adjustement : Subsystem
  Mux : Mux  Inputs=2
  Mux1 : Mux
  Right Swing leg control : Subsystem
  Stance leg control : Subsystem
  Stance leg position_initial1 : Subsystem
  Terminator : Terminator
  Terminator1 : Terminator
  Force_des : Outport
  Torques_des : Outport  Port=2  OutDataTypeStr=double  Unit=N*m
  r_vrp : Outport  Port=3
  r_extrapolated_CoM : Outport  Port=4
  Foot_adjust : Outport  Port=5
  wires:
  Stance leg control/2(Force_des) -> Force_des/1
  Stance leg control/4(r_extrapolated_CoM) -> r_extrapolated_CoM/1
  Stance leg control/3(r_vrp) -> r_vrp/1
  Stance leg control/1(Torques_des) -> Demux/1
  Mux1/1 -> Mux/2
  Mux/1 -> Torques_des/1
  Right Swing leg control/1(Torques_des) -> Mux/1
  DCM_position/1 -> Stance leg control/1(DCM_position)
  DCM_velocity/1 -> Stance leg control/2(DCM_velocity)
  joint_angle/1 -> Demux1/1
  joint_velocity/1 -> Demux2/1
  Demux1/1 -> Right Swing leg control/2(actual_joint_angle)
  Demux1/2 -> Stance leg position_initial1/1(position)
  Demux2/1 -> Right Swing leg control/4(actual_joint_velocity)
  FK_info/1 -> Martijn Step adjustement/1(FK_info), Right Swing leg control/3(FK_info), Stance leg control/3(FK_info)
  Demux2/2 -> Stance leg position_initial1/2(velocity)
  Stance leg position_initial1/1(torques) -> Demux3/1
  Demux3/3 -> Mux1/3
  Demux/2 -> Mux1/4
  Demux/1 -> Mux1/2
  Demux3/1 -> Mux1/1
  hip_trajectory/1 -> Stance leg position_initial1/3(hip_trajectory)
  Constant/1 -> Martijn Step adjustement/2(R_or_L)
  swing_state/1 -> MATLAB Function/1(swing_state)
  Martijn Step adjustement/1(StepPos) -> MATLAB Function/2(foot_adjust)
  MATLAB Function/1(new_swing_state) -> Foot_adjust/1, Right Swing leg control/1(swing_state)
  knee_trajectory/1 -> Demux4/1
  Demux4/1 -> Right Swing leg control/5(theta2)
  Demux4/2 -> Stance leg position_initial1/4(theta7)
  Demux3/2 -> Terminator/1
  Demux3/4 -> Terminator1/1

== system Control_model_10DOF_fin/Control/Stance_position/Stance control ==
  angle : Inport
  velocity : Inport  Port=2
  Constant : Constant  Value=jointsinitial
  Demux : Demux  Outputs=2
  Demux1 : Demux  Outputs=2
  Demux2 : Demux  Outputs=2
  Mux : Mux  Inputs=2
  PID left : Subsystem
  PID right : Subsystem
  Saturation1 : Saturate  UpperLimit=300  LowerLimit=-300
  Scope : Scope
  Sum : Sum  Inputs=-+|
  Sum1 : Sum  Inputs=-+|
  scope system : Subsystem
  scope system1 : Subsystem
  Torques : Outport
  wires:
  Sum/1 -> PID right/1(error)
  Mux/1 -> Saturation1/1
  Sum1/1 -> PID left/1(error)
  Saturation1/1 -> Scope/1, Torques/1
  Demux1/2 -> Sum1/1
  Demux1/1 -> Sum/1
  Demux/1 -> PID right/2(velocity)
  Demux/2 -> PID left/2(velocity)
  Demux2/1 -> Sum/2
  Demux2/2 -> Sum1/2
  PID right/1(torques_des) -> Mux/1
  PID left/1(torques_des) -> Mux/2
  Constant/1 -> scope system/1(input), Demux2/1
  angle/1 -> scope system/2(input2), Demux1/1
  velocity/1 -> scope system1/1(input), Demux/1

== system Control_model_10DOF_fin/Time//State Machine/Hip_timer/DS ==
  time : Inport
  Action Port : ActionPort  ActionType=case
  time_Hip : Outport
  wires:
  time/1 -> time_Hip/1

== system Control_model_10DOF_fin/Time//State Machine/Hip_timer/Finish_swing_phase ==
  Action Port : ActionPort  ActionType=case
  Constant : Constant  Value=0
  time_Hip : Outport
  wires:
  Constant/1 -> time_Hip/1

== system Control_model_10DOF_fin/Time//State Machine/Hip_timer/Initial_Transfert ==
  time_DS : Inport
  Action Port : ActionPort  ActionType=case
  time_Hip : Outport
  wires:
  time_DS/1 -> time_Hip/1

== system Control_model_10DOF_fin/Time//State Machine/Hip_timer/SS ==
  time_swing : Inport
  Action Port : ActionPort  ActionType=case
  First_part : Subsystem  TreatAsAtomicUnit=on
  If first part of swing : If  IfExpression=u1 <= half_time_swing
  Merge4 : Merge
  Second_part : Subsystem  TreatAsAtomicUnit=on
  time_Hip : Outport
  wires:
  time_swing/1 -> Second_part/1(time_swing), If first part of swing/1
  If first part of swing/1 -> First_part/Action
  If first part of swing/2 -> Second_part/Action
  Merge4/1 -> time_Hip/1
  Second_part/1(time_Hip) -> Merge4/2
  First_part/1(time_Hip) -> Merge4/1

== system Control_model_10DOF_fin/Time//State Machine/Hip_timer/Stance_position ==
  Action Port : ActionPort  ActionType=case
  Constant : Constant  Value=0
  time_Hip : Outport
  wires:
  Constant/1 -> time_Hip/1

== system Control_model_10DOF_fin/Trajectory generator/DCM trajectory/DS ==
  "DCM_position_ini  " : Inport  OutDataTypeStr=double  Unit=m  PortDimensions=3
  DCM_velocity_ini : Inport  Port=2  OutDataTypeStr=double  Unit=m/s  PortDimensions=3
  feet_positions : Inport  Port=3
  time : Inport  Port=4
  Action Port : ActionPort  ActionType=case
  Constant : Constant  Value=time_DS
  DCM estimate fin : MATLAB Function  TreatAsAtomicUnit=on
  DCM_points_position : MATLAB Function  TreatAsAtomicUnit=on
  MATLAB Function : MATLAB Function  TreatAsAtomicUnit=on
  Scope : Scope
  Scope x8 : Subsystem
  second_DCM : Selector  InputPortWidth=3*(nb_step-2)  IndexOptions=Index vector (dialog)  Indices=[1 2 3]  OutputSizes=1
  "second_vrp " : Selector  InputPortWidth=3*(nb_step-1)  IndexOptions=Index vector (dialog)  Indices=[1 2 3]  OutputSizes=1
  DCM_position : Outport
  DCM_velocity : Outport  Port=2
  wires:
  MATLAB Function/2(DCM_velocity) -> DCM_velocity/1
  MATLAB Function/1(DCM_position) -> DCM_position/1
  "DCM_position_ini  "/1 -> Scope x8/1(Input), MATLAB Function/1(DCM_position_ini)
  DCM_velocity_ini/1 -> MATLAB Function/2(DCM_velocity_ini)
  DCM estimate fin/1(DCM_position) -> MATLAB Function/3(DCM_position_fin)
  DCM estimate fin/2(DCM_velocity) -> MATLAB Function/4(DCM_velocity_fin)
  "second_vrp "/1 -> DCM estimate fin/1(r_vrp)
  second_DCM/1 -> DCM estimate fin/2(r_DCM)
  DCM_points_position/1(r_vrp) -> "second_vrp "/1
  DCM_points_position/2(r_DCM) -> second_DCM/1
  feet_positions/1 -> DCM_points_position/1(feet_positions)
  time/1 -> Scope/1, MATLAB Function/5(time)
  Constant/1 -> DCM estimate fin/3(time)

== system Control_model_10DOF_fin/Trajectory generator/DCM trajectory/Finish_swing_phase//SS ==
  feet_positions : Inport
  time : Inport  Port=2
  Action Port : ActionPort  ActionType=case
  Constant : Constant  Value=time_DS
  DCM trajectory generator : MATLAB Function  TreatAsAtomicUnit=on
  DCM_points_position : MATLAB Function  TreatAsAtomicUnit=on
  Sum : Sum  Inputs=|++
  "first_DCM " : Selector  InputPortWidth=3*(nb_step-2)  IndexOptions=Index vector (dialog)  Indices=[1 2 3]  OutputSizes=1
  first_vrp : Selector  InputPortWidth=3*(nb_step-1)  IndexOptions=Index vector (dialog)  Indices=[1 2 3]  OutputSizes=1
  DCM_position : Outport
  DCM_velocity : Outport  Port=2
  last_DCM_position : Outport  Port=3
  last_DCM_velocity : Outport  Port=4
  wires:
  DCM trajectory generator/2(DCM_velocity) -> last_DCM_velocity/1, DCM_velocity/1
  DCM trajectory generator/1(DCM_position) -> last_DCM_position/1, DCM_position/1
  first_vrp/1 -> DCM trajectory generator/1(r_vrp)
  "first_DCM "/1 -> DCM trajectory generator/2(r_DCM)
  DCM_points_position/2(r_DCM) -> "first_DCM "/1
  DCM_points_position/1(r_vrp) -> first_vrp/1
  feet_positions/1 -> DCM_points_position/1(feet_positions)
  Sum/1 -> DCM trajectory generator/3(time)
  Constant/1 -> Sum/2
  time/1 -> Sum/1

== system Control_model_10DOF_fin/Trajectory generator/DCM trajectory/Initial_Transfert ==
  feet_positions : Inport
  time : Inport  Port=2
  Action Port : ActionPort  ActionType=case
  CoM_position_ini : Constant  Value=initial_CoM_position
  CoM_velocity_ini : Constant  Value=[0;0;0]
  DCM_estimate_fin : Subsystem  TreatAsAtomicUnit=on
  DCM_points_position : MATLAB Function  TreatAsAtomicUnit=on
  MATLAB Function : MATLAB Function  TreatAsAtomicUnit=on
  first_DCM : Selector  InputPortWidth=3*(nb_step-2)  IndexOptions=Index vector (dialog)  Indices=[1 2 3]  OutputSizes=1
  first_vrp : Selector  InputPortWidth=3*(nb_step-1)  IndexOptions=Index vector (dialog)  Indices=[1 2 3]  OutputSizes=1
  time_IT : Constant  Value=T_IT
  DCM_position : Outport
  DCM_velocity : Outport  Port=2
  wires:
  MATLAB Function/2(DCM_velocity) -> DCM_velocity/1
  MATLAB Function/1(DCM_position) -> DCM_position/1
  DCM_estimate_fin/2(DCM_velocity) -> MATLAB Function/4(DCM_velocity_fin)
  DCM_estimate_fin/1(DCM_position) -> MATLAB Function/3(DCM_position_fin)
  time_IT/1 -> DCM_estimate_fin/3(time)
  CoM_velocity_ini/1 -> MATLAB Function/2(DCM_velocity_ini)
  CoM_position_ini/1 -> MATLAB Function/1(DCM_position_ini)
  feet_positions/1 -> DCM_points_position/1(feet_positions)
  first_vrp/1 -> DCM_estimate_fin/1(r_vrp)
  first_DCM/1 -> DCM_estimate_fin/2(r_DCM)
  DCM_points_position/1(r_vrp) -> first_vrp/1
  DCM_points_position/2(r_DCM) -> first_DCM/1
  time/1 -> MATLAB Function/5(time)

== system Control_model_10DOF_fin/Trajectory generator/DCM trajectory/Stance_position ==
  Action Port : ActionPort  ActionType=case
  CoM_position_ini : Constant  Value=initial_CoM_position
  CoM_velocity_ini : Constant  Value=[0;0;0]
  DCM_position : Outport
  DCM_velocity : Outport  Port=2
  wires:
  CoM_velocity_ini/1 -> DCM_velocity/1
  CoM_position_ini/1 -> DCM_position/1

== system Control_model_10DOF_fin/Trajectory generator/Enabled and Triggered Subsystem 1/Feet Pattern generator ==
  Constant : Constant  Value=initial_RorL
  Pattern creator : MATLAB Function  TreatAsAtomicUnit=on
  initial position : Subsystem  TreatAsAtomicUnit=on
  Feet_pattern : Outport
  wires:
  initial position/1(initial_swing_foot) -> Pattern creator/1(swing_foot_position)
  initial position/2(initial_stance_foot) -> Pattern creator/2(stance_foot_position)
  Constant/1 -> Pattern creator/3(RorL)
  Pattern creator/1(feet_positions) -> Feet_pattern/1

== system Control_model_10DOF_fin/Trajectory generator/Enabled and Triggered Subsystem 1/initial position ==
  Action Port : ActionPort  ActionType=case
  Constant : Constant  Value=initial_RorL
  If first right swing : If  IfExpression=u1 ==1
  Merge1 : Merge
  Merge2 : Merge
  initial position : Subsystem  TreatAsAtomicUnit=on
  initial position1 : Subsystem  TreatAsAtomicUnit=on
  initial_swing_foot : Outport
  initial_stance_foot : Outport  Port=2  PortDimensions=3
  wires:
  If first right swing/1 -> initial position/Action
  If first right swing/2 -> initial position1/Action
  initial position/1(initial_swing_foot) -> Merge1/1
  initial position/2(initial_stance_foot) -> Merge2/1
  Merge1/1 -> initial_swing_foot/1
  Merge2/1 -> initial_stance_foot/1
  Constant/1 -> If first right swing/1
  initial position1/1(initial_swing_foot) -> Merge1/2
  initial position1/2(initial_stance_foot) -> Merge2/2

== system Control_model_10DOF_fin/Trajectory generator/Enabled and Triggered Subsystem 1/initial position1 ==
  FK_info : Inport
  RorL : Inport  Port=2
  Action Port : ActionPort  ActionType=case
  Bus Selector : BusSelector  OutputSignals=TWR,TWL
  If Right swing phase : If  IfExpression=u1 ==1
  Left : Subsystem  TreatAsAtomicUnit=on
  Merge1 : Merge
  Merge2 : Merge
  Right : Subsystem  TreatAsAtomicUnit=on
  initial_swing_foot : Outport  PortDimensions=3
  initial_stance_foot : Outport  Port=2  PortDimensions=3
  wires:
  FK_info/1 -> Bus Selector/1
  RorL/1 -> If Right swing phase/1
  If Right swing phase/1 -> Right/Action
  If Right swing phase/2 -> Left/Action
  Merge2/1 -> initial_swing_foot/1
  Merge1/1 -> initial_stance_foot/1
  Right/1(initial_swing_foot) -> Merge2/1
  Left/1(initial_swing_foot) -> Merge2/2
  Right/2(initial_stance_foot) -> Merge1/1
  Left/2(initial_stance_foot) -> Merge1/2
  Bus Selector/1 -> Left/1(Right_foot), Right/1(Right_foot)  "<TWR>"
  Bus Selector/2 -> Right/2(Left_foot), Left/2(Left_foot)  "<TWL>"

== system Control_model_10DOF_fin/Trajectory generator/Enabled and Triggered Subsystem 1/initial position2 ==
  FK_info : Inport
  RorL : Inport  Port=2
  Action Port : ActionPort  ActionType=case
  Bus Selector : BusSelector  OutputSignals=TWR,TWL
  If Right swing phase : If  IfExpression=u1 ==1
  Left : Subsystem  TreatAsAtomicUnit=on
  Merge1 : Merge
  Merge2 : Merge
  Right : Subsystem  TreatAsAtomicUnit=on
  initial_swing_foot : Outport  PortDimensions=3
  initial_stance_foot : Outport  Port=2  PortDimensions=3
  wires:
  FK_info/1 -> Bus Selector/1
  RorL/1 -> If Right swing phase/1
  If Right swing phase/1 -> Right/Action
  If Right swing phase/2 -> Left/Action
  Merge2/1 -> initial_swing_foot/1
  Merge1/1 -> initial_stance_foot/1
  Right/1(initial_swing_foot) -> Merge2/1
  Left/1(initial_swing_foot) -> Merge2/2
  Right/2(initial_stance_foot) -> Merge1/1
  Left/2(initial_stance_foot) -> Merge1/2
  Bus Selector/1 -> Left/1(Right_foot), Right/1(Right_foot)  "<TWR>"
  Bus Selector/2 -> Right/2(Left_foot), Left/2(Left_foot)  "<TWL>"

== system Control_model_10DOF_fin/Trajectory generator/Enabled and Triggered Subsystem 1/selector ==
  In1 : Inport
  nb_step : Inport  Port=2
  1 : Subsystem
  2 : Subsystem
  3 : Subsystem
  Mux : Mux  Inputs=3
  Variable Selector : dspindex/Variable Selector  NumInputs=1  rowsOrCols=Rows  IdxMode=Variable  Elements=[1 3]  ZerOneIdxMode=One-based  errmode=Clip Index  FillMode=on  FillValues=0
  Variable Selector1 : dspindex/Variable Selector  NumInputs=1  rowsOrCols=Rows  IdxMode=Variable  Elements=[1 3]  ZerOneIdxMode=One-based  errmode=Clip Index  FillMode=on  FillValues=0
  Variable Selector2 : dspindex/Variable Selector  NumInputs=1  rowsOrCols=Rows  IdxMode=Variable  Elements=[1 3]  ZerOneIdxMode=One-based  errmode=Clip Index  FillMode=on  FillValues=0
  Out1 : Outport
  wires:
  In1/1 -> Variable Selector2/1, Variable Selector1/1, Variable Selector/1
  Mux/1 -> Out1/1
  Variable Selector/1 -> Mux/1
  Variable Selector1/1 -> Mux/2
  Variable Selector2/1 -> Mux/3
  nb_step/1 -> 1/1(In1), 3/1(In1), 2/1(In1)
  1/1(Out1) -> Variable Selector/2
  2/1(Out1) -> Variable Selector1/2
  3/1(Out1) -> Variable Selector2/2
